simulink model "systune_gain_scheduling_darko"  (R2021b)
settings: Solver=VariableStepAuto  StartTime=0.0  StopTime=100  RelTol=1e-3
values from neighbouring files (symbols this model uses):
  C_control = [C(1:7,:);C(9:12,:)]    [systune_constant_gain_LPV.m]    (also in systune_gain_scheduling.m; systune_variable_gain_scheduling_LPV.m)
  drone = struct('MASS',               0.492,                      'INERTIA',            eye(3),                     'G',                  9.81,                       'P_P1_CG',            [1; 1; 1],                  'P_P2_CG',            [1; 1; 1],                  'P_A1_CG',            [1; 1; 1],                  'P_A2_CG',            [1; 1; 1],                  'INERTIA_PROP_X',     5.1116e-6,            ...(+949 chars)    [generateDarko.m]    (also in systune_constant_gain_LPV.m = generateDarko(); systune_gain_scheduling.m = generateDarko(); systune_variable_gain_scheduling_LPV.m = generateDarko())
  H_InputOffset = H.Normalization.InputOffset    [systune_variable_gain_scheduling_LPV.m]
  H_InputScaling = H.Normalization.InputScaling    [systune_variable_gain_scheduling_LPV.m]
  H_val = [0.174893532101 -0.170983587428 0.116298770163 -0.120491253945 -0.591123259979 0.466999830321 0.606251408925 -0.36729072329 0.527922365719 -0.579504209683 -0.860165616929 0.217648206511 ... (22 elements, 2x11)]    [matrix.mat]    (also in systune_constant_gain_LPV.m = H_val.D; systune_gain_scheduling.m = H_val.D; systune_variable_gain_scheduling_LPV.m = getBlockValue(T,'H'))
  initial_state = [p_initial; v_initial; q_initial; omega_initial]    [systune_constant_gain_LPV.m]    (also in systune_gain_scheduling.m; systune_variable_gain_scheduling_LPV.m)
  K_InputOffset = K.Normalization.InputOffset    [systune_variable_gain_scheduling_LPV.m]
  K_InputScaling = K.Normalization.InputScaling    [systune_variable_gain_scheduling_LPV.m]
  K_val = [-0.717823721707 -0.535586914826 0.293461018845 0.259857970212 -0.116645066118 0.0068635572033 0.0510701432383 0.0105656377564 -0.103136434688 -0.470758687236 -0.215457393556 0.229494669048 ... (44 elements, 4x11)]    [matrix.mat]    (also in systune_constant_gain_LPV.m = K_val.D; systune_gain_scheduling.m = K_val.D; systune_variable_gain_scheduling_LPV.m = getBlockValue(T,'K'))
  u_eq = [2.43630788633 2.43630788633 0 0]    [matrix.mat]    (also in matrix_lqr.mat = [1.98073811897 1.98073811897 0 0]; systune_constant_gain_LPV.m = [ua;ua;ub;ub]; systune_gain_scheduling.m = [ua;ua;ub;ub]; systune_variable_gain_scheduling_LPV.m = [ua;ua;ub;ub])
  w = [-i*0.4;0;0]    [systune_constant_gain_LPV.m]    (also in systune_gain_scheduling.m = [0;0;0]; systune_variable_gain_scheduling_LPV.m = [-i;0;0])
  x_eq_ = [0 0 0 0 0 0 0 0 0 0 0]    [matrix.mat]    (also in matrix_lqr.mat; systune_constant_gain_LPV.m = [[0; 0; 0]; [0; 0; 0]; [0; 0]; [0; 0; 0]]; systune_gain_scheduling.m = [[0; 0; 0]; [0; 0; 0]; [0; 0]; [0; 0; 0]]; systune_variable_gain_scheduling_LPV.m = [[0; 0; 0]; [0; 0; 0]; [0; 0]; [0; 0; 0]])
libraries: simulink_extras x7, aerolibanim x1, sharedtransform x1
settings Model: Creator=florian  LastModifiedBy=florian
settings SolverCC: AlgebraicLoopSolver=TrustRegion
settings DebuggingCC: SFMachineParentedDataDiag=warning

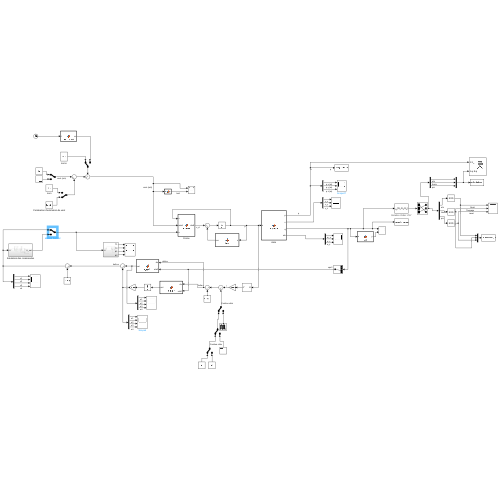
[thumbnail: Simulink's stored preview of the top-level diagram]
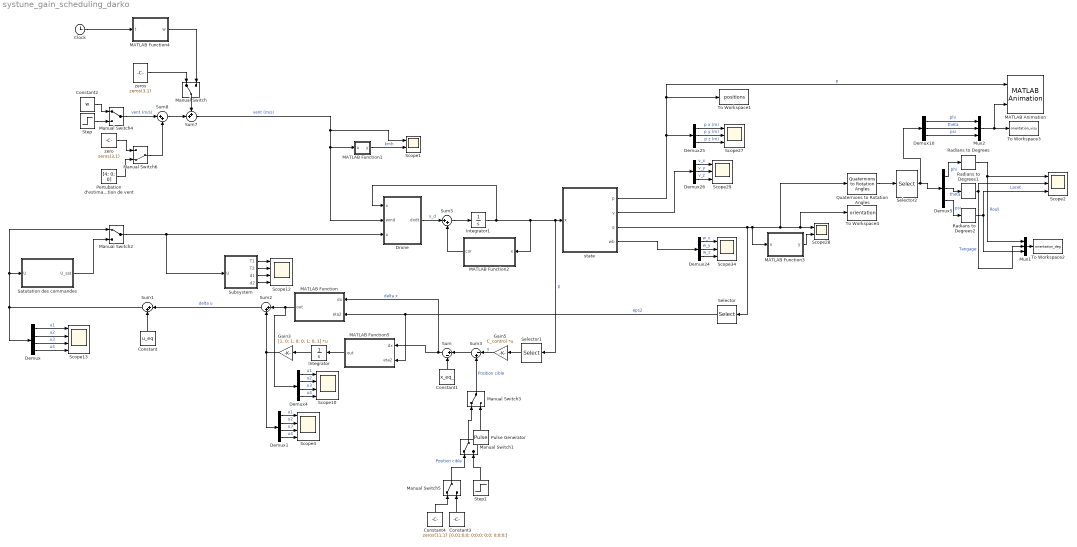
== system systune_gain_scheduling_darko ==
  Clock : Clock
  Constant : Constant  Value=u_eq
  Constant1 : Constant  Value=x_eq_
  Constant2 : Constant  Value=w
  Constant3 : Constant  Value=[0.01;0;0; 0;0;0; 0;0; 0;0;0;]
  Constant4 : Constant  Value=zeros(11,1)
  Demux : Demux
  Demux1 : Demux
  Demux{5,10,24..26} (5 alike) : Demux  Outputs=3
  Demux4 : Demux
  Drone : MATLAB Function  TreatAsAtomicUnit=on
  Gain3 : Gain  Gain=[1, 0; 1, 0; 0, 1; 0, 1]  Multiplication=Matrix(K*u) (u vector)
  Gain5 : Gain  Gain=C_control  Multiplication=Matrix(K*u) (u vector)
  Integrator : Integrator
  Integrator1 : Integrator  InitialCondition=initial_state
  MATLAB Animation : aerolibanim/MATLAB Animation  Tag=Matlab Animation 6 DOF  Vehicles=1  Geometries='astredwedge.mat'  BoundingBoxCoordinates=[-50,50,-50,50,-50,50]  CameraOffset=[0,-50,0]  CameraViewAngle=10  SampleTime=0.08  FigurePosition=[635,-23,492,413]
      settings: SourceProductBaseCode=AE
  MATLAB Function : MATLAB Function  TreatAsAtomicUnit=on
  MATLAB Function1 : MATLAB Function  TreatAsAtomicUnit=on
  MATLAB Function2 : MATLAB Function  TreatAsAtomicUnit=on
  MATLAB Function3 : MATLAB Function  TreatAsAtomicUnit=on
  MATLAB Function4 : MATLAB Function  TreatAsAtomicUnit=on
  MATLAB Function5 : MATLAB Function  TreatAsAtomicUnit=on
  Manual Switch{,1..5} (6 alike) : ManualSwitch
  Manual Switch6 : ManualSwitch  CurrentSetting=0
  Mux1 : Mux  Inputs=3
  Mux2 : Mux  Inputs=3
  Pertubation d'estimation de vent : Constant  Value=[4; 0; 0]
  Pulse Generator : DiscretePulseGenerator  PulseType=Time based  Amplitude=[0;0;-5; 0;0;0; 0;0; 0;0;0]  Period=5  PulseWidth=50
  Quaternions to Rotation Angles : sharedtransform/Quaternions to Rotation Angles  rotationOrder=ZXY  aMode=aMode
      settings: SourceProductBaseCode=AE,PW,DR,MT,UV,VE
  Radians to Degrees : simulink_extras/Transformations/Radians to Degrees
  Radians to Degrees1 : simulink_extras/Transformations/Radians to Degrees
  Radians to Degrees2 : simulink_extras/Transformations/Radians to Degrees
  Satutation des commandes : Subsystem
  Scope1 : Scope  NumInputPorts=2
  Scope{4,10,12..13} (4 alike) : Scope  NumInputPorts=4
  Scope{2,27,29,34} (4 alike) : Scope  NumInputPorts=3
  Scope28 : Scope  NumInputPorts=2
  Selector : Selector  InputPortWidth=4  IndexOptions=Index vector (dialog)  Indices=[3]  OutputSizes=1
  Selector1 : Selector  InputPortWidth=13  IndexOptions=Index vector (dialog)  Indices=[1:6 8:13]  OutputSizes=1
  Selector2 : Selector  InputPortWidth=3  IndexOptions=Index vector (dialog)  Indices=[2 3 1]  OutputSizes=1
  Step : Step  Time=20  Before=[0;0;0]  After=[-7;0;0]  SampleTime=0
  Step1 : Step  Time=35  Before=zeros(11,1)  After=[-0.1;0;0; 0;0;0; 0;0; 0;0;0]  SampleTime=0
  Subsystem : Subsystem
  Sum : Sum  Inputs=|+-
  Sum{1..2,5,8} (4 alike) : Sum  Inputs=|++
  Sum3 : Sum  Inputs=|-+
  Sum7 : Sum  Inputs=++|
  To Workspace1 : ToWorkspace  VariableName=positions  SampleTime=-1
  To Workspace2 : ToWorkspace  VariableName=orientation_deg  SampleTime=-1
  To Workspace3 : ToWorkspace  VariableName=orientation_visu  SampleTime=-1
  To Workspace4 : ToWorkspace  VariableName=orientation  SampleTime=-1
  state : MATLAB Function  TreatAsAtomicUnit=on
  zero : Constant  Value=zeros(3,1)
  zeros : Constant  Value=zeros(3,1)
  wires:
  Sum5/1 -> Integrator1/1
  MATLAB Function2/1(cor) -> Sum5/2
  Drone/1(dxdt) -> Sum5/1  "x_d"
  Demux25/3 -> Scope27/3  "p z (m)"
  Demux26/2 -> Scope29/2  "v_y"
  Demux24/1 -> Scope34/1  "w_x"
  MATLAB Function3/1(y) -> Scope28/2
  Demux25/1 -> Scope27/1  "p x (m)"
  state/4(wb) -> Demux24/1
  Demux24/2 -> Scope34/2  "w_y"
  Demux24/3 -> Scope34/3  "w_z"
  state/2(v) -> Demux26/1
  Demux25/2 -> Scope27/2  "p y (m)"
  Demux26/3 -> Scope29/3  "v_z"
  Demux26/1 -> Scope29/1  "v_x"
  Constant1/1 -> Sum/2
  Demux5/2 -> Radians to Degrees1/1  "theta"
  Demux5/1 -> Radians to Degrees/1  "phi"
  Demux5/3 -> Radians to Degrees2/1  "psi"
  Demux/3 -> Scope13/3  "u3"
  Sum1/1 -> Demux/1, Satutation des commandes/1(U), Manual Switch2/1
  Demux/2 -> Scope13/2  "u2"
  Demux/1 -> Scope13/1  "u1"
  Demux/4 -> Scope13/4  "u4"
  Mux1/1 -> To Workspace2/1
  state/3(q) -> Quaternions to Rotation Angles/1, Scope28/1, To Workspace4/1, MATLAB Function3/1(u), Selector/1
  Satutation des commandes/1(U_sat) -> Manual Switch2/2
  Demux10/2 -> Mux2/2  "theta"
  Selector2/1 -> Demux10/1, Demux5/1
  Demux10/1 -> Mux2/1  "phi"
  Demux10/3 -> Mux2/3  "psi"
  state/1(p) -> Demux25/1, MATLAB Animation/1, To Workspace1/1  "p"
  Mux2/1 -> To Workspace3/1, MATLAB Animation/2
  Sum7/1 -> Drone/2(wind), MATLAB Function1/1(u), Scope1/1  "vent (m/s)"
  Radians to Degrees1/1 -> Mux1/2, Scope2/2  "Tangage"
  Radians to Degrees/1 -> Scope2/1, Mux1/1  "Rouli"
  Radians to Degrees2/1 -> Scope2/3, Mux1/3  "Lacet"
  Integrator/1 -> Gain3/1
  Sum/1 -> MATLAB Function5/1(dx), MATLAB Function/1(dx)  "delta x"
  MATLAB Function5/1(out) -> Integrator/1
  MATLAB Function/1(out) -> Demux4/1, Sum2/1
  Demux1/2 -> Scope4/2  "u2"
  Demux1/3 -> Scope4/3  "u3"
  Demux1/4 -> Scope4/4  "u4"
  Demux1/1 -> Scope4/1  "u1"
  Selector1/1 -> Gain5/1
  Gain5/1 -> Sum3/1  "y"
  Sum3/1 -> Sum/1
  Gain3/1 -> Sum2/2, Demux1/1
  Demux4/2 -> Scope10/2  "u2"
  Demux4/3 -> Scope10/3  "u3"
  Demux4/4 -> Scope10/4  "u4"
  Demux4/1 -> Scope10/1  "u1"
  Step/1 -> Manual Switch4/2
  Constant2/1 -> Manual Switch4/1
  MATLAB Function1/1(y) -> Scope1/2  "kmh"
  Step1/1 -> Manual Switch1/2
  Pulse Generator/1 -> Manual Switch3/2
  Manual Switch1/1 -> Manual Switch3/1
  Manual Switch3/1 -> Sum3/2  "Position cible"
  Quaternions to Rotation Angles/1 -> Selector2/1
  Clock/1 -> MATLAB Function4/1(t)
  Constant3/1 -> Manual Switch5/2
  Manual Switch5/1 -> Manual Switch1/1  "Position cible"
  Constant4/1 -> Manual Switch5/1
  Integrator1/1 -> Drone/1(x), Selector1/1, state/1(x), MATLAB Function2/1(x)  "p"
  Subsystem/1(T1) -> Scope12/1
  Subsystem/3(d1) -> Scope12/3
  Manual Switch2/1 -> Drone/3(u), Subsystem/1(U)
  Subsystem/2(T2) -> Scope12/2
  Subsystem/4(d2) -> Scope12/4
  Manual Switch/1 -> Sum7/1
  MATLAB Function4/1(w) -> Manual Switch/2
  zeros/1 -> Manual Switch/1
  Sum8/1 -> Sum7/2
  Manual Switch4/1 -> Sum8/1  "vent (m/s)"
  Pertubation d'estimation de vent/1 -> Manual Switch6/2
  Manual Switch6/1 -> Sum8/2
  zero/1 -> Manual Switch6/1
  Constant/1 -> Sum1/2
  Sum2/1 -> Sum1/1  "delta u"
  Selector/1 -> MATLAB Function5/2(eta2), MATLAB Function/2(eta2)  "eps2"

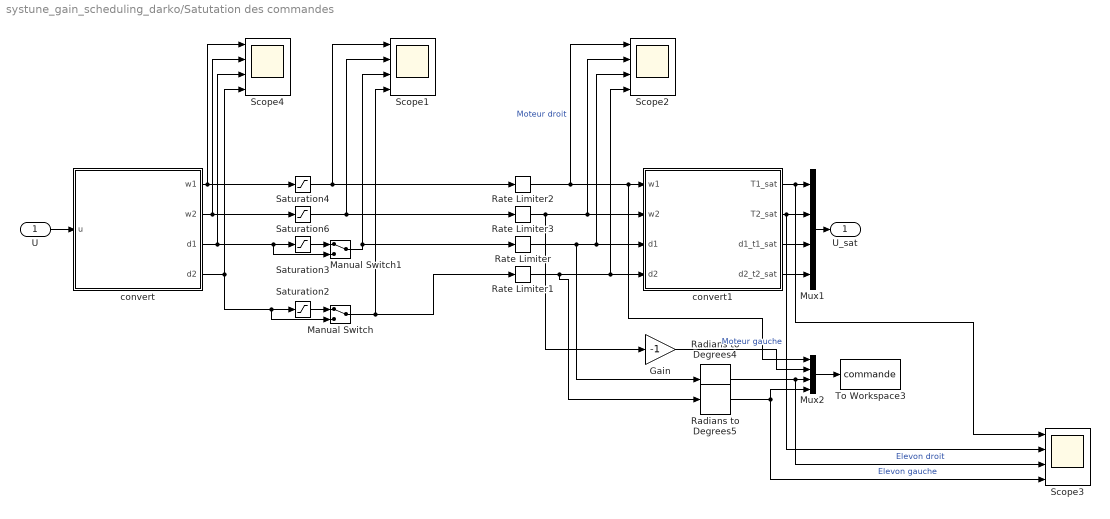
== system systune_gain_scheduling_darko/Satutation des commandes ==
  U : Inport
  Gain : Gain  Gain=-1
  Manual Switch : ManualSwitch
  Manual Switch1 : ManualSwitch
  Mux1 : Mux
  Mux2 : Mux
  Radians to Degrees4 : simulink_extras/Transformations/Radians to Degrees
  Radians to Degrees5 : simulink_extras/Transformations/Radians to Degrees
  Rate Limiter : RateLimiter  RisingSlewLimit=drone.ELEVON_RATE_CHANGE  FallingSlewLimit=-drone.ELEVON_RATE_CHANGE  SampleTimeMode=inherited
  Rate Limiter1 : RateLimiter  RisingSlewLimit=drone.ELEVON_RATE_CHANGE  FallingSlewLimit=-drone.ELEVON_RATE_CHANGE  SampleTimeMode=inherited
  Rate Limiter2 : RateLimiter  RisingSlewLimit=drone.MOTOR_RATE_CHANGE  FallingSlewLimit=-drone.MOTOR_RATE_CHANGE  SampleTimeMode=inherited
  Rate Limiter3 : RateLimiter  RisingSlewLimit=drone.MOTOR_RATE_CHANGE  FallingSlewLimit=-drone.MOTOR_RATE_CHANGE  SampleTimeMode=inherited
  Saturation2 : Saturate  UpperLimit=30*(pi/180)  LowerLimit=-30*(pi/180)
  Saturation3 : Saturate  UpperLimit=30*(pi/180)  LowerLimit=-30*(pi/180)
  Saturation4 : Saturate  UpperLimit=1000  LowerLimit=200
  Saturation6 : Saturate  UpperLimit=1000  LowerLimit=200
  Scope{1..4} (4 alike) : Scope  NumInputPorts=4
  To Workspace3 : ToWorkspace  VariableName=commande  SampleTime=-1
  convert : MATLAB Function  TreatAsAtomicUnit=on
  convert1 : MATLAB Function  TreatAsAtomicUnit=on
  U_sat : Outport
  wires:
  convert/1(w1) -> Saturation4/1, Scope4/1
  convert/2(w2) -> Scope4/2, Saturation6/1
  convert/3(d1) -> Scope4/3, Manual Switch1/2, Saturation3/1
  convert/4(d2) -> Manual Switch/2, Saturation2/1, Scope4/4
  convert1/1(T1_sat) -> Scope3/1, Mux1/1
  convert1/4(d2_t2_sat) -> Mux1/4
  Mux1/1 -> U_sat/1
  convert1/2(T2_sat) -> Scope3/2, Mux1/2
  convert1/3(d1_t1_sat) -> Mux1/3
  Saturation6/1 -> Rate Limiter3/1, Scope1/2
  Saturation4/1 -> Rate Limiter2/1, Scope1/1
  U/1 -> convert/1(u)
  Radians to Degrees5/1 -> Mux2/4, Scope3/4  "Elevon gauche"
  Rate Limiter3/1 -> Gain/1, convert1/2(w2), Scope2/2
  Rate Limiter1/1 -> Radians to Degrees5/1, Scope2/4, convert1/4(d2)
  Rate Limiter/1 -> Radians to Degrees4/1, Scope2/3, convert1/3(d1)
  Gain/1 -> Mux2/2  "Moteur gauche"
  Mux2/1 -> To Workspace3/1
  Radians to Degrees4/1 -> Scope3/3, Mux2/3  "Elevon droit"
  Rate Limiter2/1 -> Scope2/1, Mux2/1, convert1/1(w1)  "Moteur droit"
  Saturation3/1 -> Manual Switch1/1
  Manual Switch1/1 -> Rate Limiter/1, Scope1/3
  Saturation2/1 -> Manual Switch/1
  Manual Switch/1 -> Scope1/4, Rate Limiter1/1

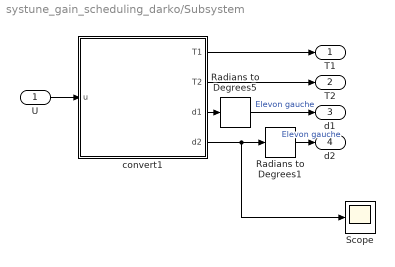
== system systune_gain_scheduling_darko/Subsystem ==
  U : Inport
  Radians to Degrees1 : simulink_extras/Transformations/Radians to Degrees
  Radians to Degrees5 : simulink_extras/Transformations/Radians to Degrees
  Scope : Scope
  convert1 : MATLAB Function  TreatAsAtomicUnit=on
  T1 : Outport
  T2 : Outport  Port=2
  d1 : Outport  Port=3
  d2 : Outport  Port=4
  wires:
  U/1 -> convert1/1(u)
  convert1/1(T1) -> T1/1
  convert1/2(T2) -> T2/1
  Radians to Degrees5/1 -> d1/1  "Elevon gauche"
  convert1/3(d1) -> Radians to Degrees5/1
  Radians to Degrees1/1 -> d2/1  "Elevon gauche"
  convert1/4(d2) -> Scope/1, Radians to Degrees1/1

== matlab function systune_gain_scheduling_darko/MATLAB Function3 ==
  data: u input; y output
function y = fcn(u)
%#codegen

y = norm(u);

== matlab function systune_gain_scheduling_darko/state ==
  data: x input; p output; v output; q output; wb output
function [p, v, q, wb] = demux(x)
%#codegen

p = x(1:3);
v = x(4:6);
q  = x(7:10);
wb = x(11:13);

== matlab function systune_gain_scheduling_darko/MATLAB Function ==
  data: dx input; eta2 input; out output; K_val parameter; K_InputOffset parameter; K_InputScaling parameter
function out = K_gain(dx, eta2, K_val, K_InputOffset, K_InputScaling)

n_eta2 = (eta2 - K_InputOffset)/K_InputScaling;

% K = K_val(:,1:11) + K_val(:,12:22)*n_eta2 +  K_val(:,23:33)*n_eta2^2;
K = K_val(:,1:11) + K_val(:,12:22)*n_eta2;

out = K*dx;

== matlab function systune_gain_scheduling_darko/Drone ==
  data: x input; wind input; u input; dxdt output; drone parameter
function dxdt  = drone(x,wind, u, drone)

%% physical constants
% gravity
g = drone.G;
% vehicle mass
m = drone.MASS;
% vehicle inertia matrix
J = drone.INERTIA; % [3x3 real symmetric] in body axis

%% state demultiplexing
% p = x(1:3);
v = x(4:6);
q  = x(7:10);
wb = x(11:13);

Rq = q2dcm(q);

[Fp, Mp] = external_force_moment(x, u, wind, drone);

% position
dpdt = v;

% kinematics
dvdt =  [0;0;g] + (1/m)*Rq*drone.Fb*u + (1/m)*Rq*Fp; 

%% quaternion derivative
eta = q(1);
eps = q(2:4);

dqdt = (1/2)*[-eps'; eta*eye(3) + skew_sym(eps)]*wb;

%% angular velocity derivative
% kinematics
dwdt = -J\cross(wb, J*wb) + J\(drone.Mb*u) + J\Mp;


%% derivative multiplexing
dxdt = [dpdt; dvdt; dqdt; dwdt] ;

== matlab function systune_gain_scheduling_darko/Subsystem/convert1 ==
  data: u input; T1 output; drone parameter; T2 output; d1 output; d2 output
function [T1, T2, d1, d2] = convert(u, drone)
%#codegen
kf = drone.PROP_KP;

T1 = max(u(1),0);
T2 = max(u(2),0);
d1_T1 = u(3);
d2_T2 = u(4);

w1 = sqrt(T1/kf);
w2 = sqrt(T2/kf);
d1 = d1_T1/T1;
d2 = d2_T2/T2;

== matlab function systune_gain_scheduling_darko/MATLAB Function1 ==
  data: u input; y output
function y = nor(u)
%#codegen

y = norm(u)*3.6;

== matlab function systune_gain_scheduling_darko/MATLAB Function4 ==
  data: t input; w output
function w = mex_wind(t)
%#codegen
t0 = 60; %s
wx_mean = 0;
fg = 0.8;
Ag = -1; %m/s
if (t-t0)<0 ||  (t-t0)> 1/fg
    wx = wx_mean;
else
    wx = wx_mean + (Ag/2)*(1-cos(2*pi*fg*(t-t0)))*sin(3*pi*fg*(t-t0));
end
w = [-wx;0;0];

== matlab function systune_gain_scheduling_darko/MATLAB Function5 ==
  data: dx input; eta2 input; out output; H_val parameter; H_InputOffset parameter; H_InputScaling parameter
function out = H_gain(dx, eta2, H_val, H_InputOffset, H_InputScaling)



n_eta2 = (eta2 - H_InputOffset)/H_InputScaling;

% H = H_val(:,1:11) + H_val(:,12:22)*n_eta2 +  H_val(:,23:33)*n_eta2^2;
H = H_val(:,1:11) + H_val(:,12:22)*n_eta2;

out = H*dx;

== matlab function systune_gain_scheduling_darko/Satutation des commandes/convert ==
  data: u input; w1 output; drone parameter; w2 output; d1 output; d2 output
function [w1, w2, d1, d2] = convert(u, drone)
%#codegen
kf = drone.PROP_KP;

T1 = max(u(1),0);
T2 = max(u(2),0);
d1 = u(3);
d2 = u(4);

w1 = sqrt(T1/kf);
w2 = sqrt(T2/kf);

== matlab function systune_gain_scheduling_darko/Satutation des commandes/convert1 ==
  data: w1 input; w2 input; d1 input; d2 input; T1_sat output; T2_sat output; drone parameter; d1_t1_sat output; d2_t2_sat output
function [T1_sat, T2_sat, d1_t1_sat, d2_t2_sat] = convert2(w1, w2, d1, d2, drone)
%#codegen
kf = drone.PROP_KP;

T1_sat = kf*w1^2;
d1_t1_sat = d1*T1_sat;
T2_sat = kf*w2^2;
d2_t2_sat = d2*T2_sat;

== matlab function systune_gain_scheduling_darko/MATLAB Function2 ==
  data: x input; cor output
function cor  = fcn(x)
%#codegen
q  = x(7:10);
n = norm(q);
mismatch = 1-n;
cor = [0;0;0; 0;0;0; mismatch*q; 0;0;0];
